simulink model "controller"  (R2024b)
settings: Solver=FixedStepAuto  StartTime=0.0  StopTime=8  FixedStep=0.025  RelTol=1e-3
values from neighbouring files (symbols this model uses):
  DryMass = 3    [FlightPathGeneration.m]
  LaunchSitePressure = PlanMeta(7)    [FlightAnalysis.m]    (also in FlightPathGeneration.m = 101325; TargetApogeeSelection.m = 101325)
  LaunchSiteTemperature = PlanMeta(6)    [FlightAnalysis.m]    (also in FlightPathGeneration.m = 288.15; TargetApogeeSelection.m = 288.15)
  MaximumDragArea = 0.01    [FlightPathGeneration.m]    (also in TargetApogeeSelection.m)
  MinimumDragArea = 0.0025    [FlightPathGeneration.m]    (also in TargetApogeeSelection.m)
undefined symbols (not defined in the file or in its folder): SimAngleSamples, SimMesh, SimVelocitySamples
settings Model: Creator=natha  LastModifiedBy=natha

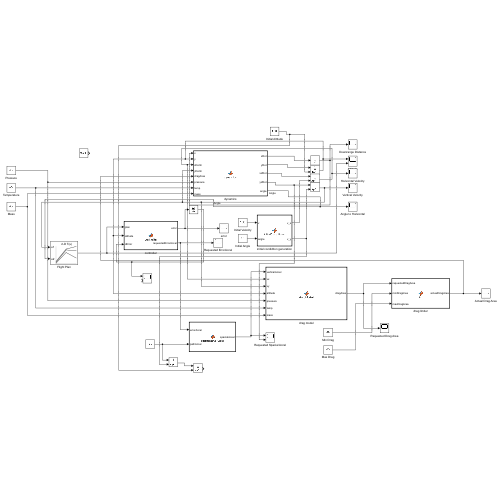
[thumbnail: Simulink's stored preview of the top-level diagram]
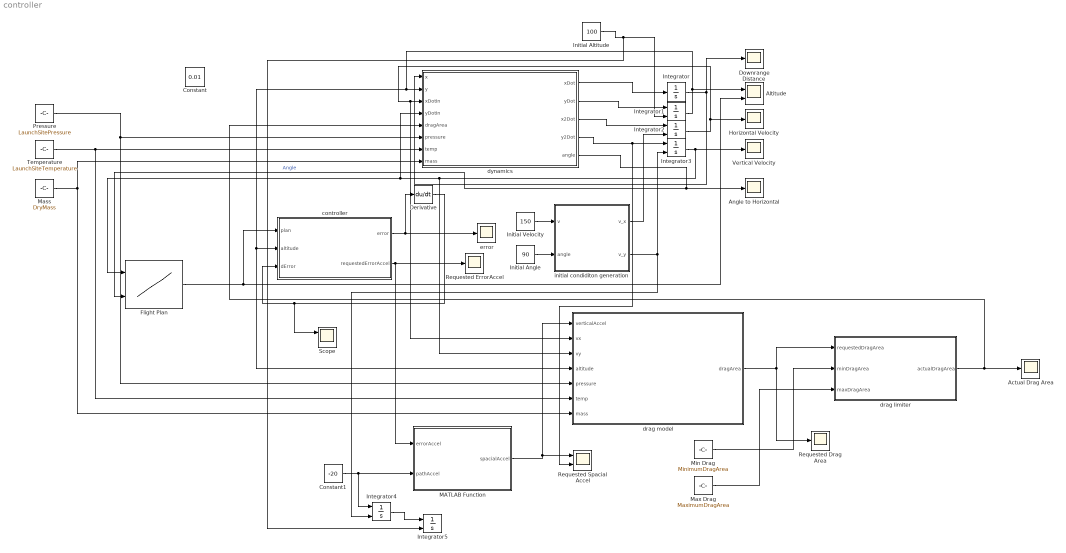
== system controller ==
  Actual Drag Area : Scope
  Altitude : Scope  NumInputPorts=2
  Angle to Horizontal : Scope
  Constant : Constant  Value=0.01
  Constant1 : Constant  Value=-20
  Derivative : Derivative
  Downrange Distance : Scope
  Flight Plan : Lookup_n-D  BreakpointsForDimension1=SimVelocitySamples  BreakpointsForDimension2=SimAngleSamples  Table=SimMesh  InternalRulePriority=Speed  RndMeth=Simplest
      settings: InputPortMap=u0,u1
  Horizontal Velocity : Scope
  Initial Altitude : Constant  Value=100
  Initial Angle : Constant  Value=90
  Initial Velocity : Constant  Value=150
  Integrator : Integrator
  Integrator{1..5} (5 alike) : Integrator  InitialConditionSource=external
  MATLAB Function : MATLAB Function  TreatAsAtomicUnit=on
  Mass : Constant  Value=DryMass
  Max Drag : Constant  Value=MaximumDragArea
  Min Drag : Constant  Value=MinimumDragArea
  Pressure : Constant  Value=LaunchSitePressure
  Requested Drag Area : Scope
  Requested ErrorAccel : Scope
  Requested Spacial Accel : Scope  NumInputPorts=2
  Scope : Scope  NumInputPorts=2
  Temperature : Constant  Value=LaunchSiteTemperature
  Vertical Velocity : Scope
  controller : MATLAB Function  TreatAsAtomicUnit=on
  drag limiter : MATLAB Function  TreatAsAtomicUnit=on
  drag model : MATLAB Function  TreatAsAtomicUnit=on
  dynamics : MATLAB Function  TreatAsAtomicUnit=on
  error : Scope
  initial condiditon generation : MATLAB Function  TreatAsAtomicUnit=on
  wires:
  dynamics/1(xDot) -> Integrator/1
  dynamics/2(yDot) -> Integrator1/1
  dynamics/3(x2Dot) -> Integrator2/1
  dynamics/4(y2Dot) -> Requested Spacial Accel/2, Integrator3/1
  Integrator/1 -> Downrange Distance/1, dynamics/1(x)
  Integrator1/1 -> drag model/4(altitude), controller/2(altitude), dynamics/2(y), Altitude/1
  Integrator2/1 -> drag model/2(vx), dynamics/3(xDotIn), Horizontal Velocity/1
  Integrator3/1 -> Flight Plan/1, dynamics/4(yDotIn), drag model/3(vy), Vertical Velocity/1
  Initial Velocity/1 -> initial condiditon generation/1(v)
  Initial Angle/1 -> initial condiditon generation/2(angle)
  initial condiditon generation/1(v_x) -> Integrator2/2
  initial condiditon generation/2(v_y) -> Integrator3/2, Integrator4/2
  Initial Altitude/1 -> Integrator5/2, Integrator1/2
  dynamics/5(angle) -> Flight Plan/2, Angle to Horizontal/1  "Angle"
  controller/1(error) -> error/1, Derivative/1
  drag model/1(dragArea) -> Requested Drag Area/1, drag limiter/1(requestedDragArea)
  Pressure/1 -> drag model/5(pressure), dynamics/6(pressure)
  Temperature/1 -> drag model/6(temp), dynamics/7(temp)
  drag limiter/1(actualDragArea) -> dynamics/5(dragArea), Actual Drag Area/1
  Mass/1 -> drag model/7(mass), dynamics/8(mass)
  MATLAB Function/1(spacialAccel) -> drag model/1(verticalAccel), Requested Spacial Accel/1
  controller/2(requestedErrorAccel) -> MATLAB Function/1(errorAccel), Requested ErrorAccel/1
  Min Drag/1 -> drag limiter/2(minDragArea)
  Max Drag/1 -> drag limiter/3(maxDragArea)
  Constant1/1 -> Integrator4/1, MATLAB Function/2(pathAccel)
  Integrator4/1 -> Integrator5/1
  Derivative/1 -> Scope/1, controller/3(dError)
  Flight Plan/1 -> Altitude/2, controller/1(plan)

== matlab function controller/initial condiditon generation ==
  data: v input; v_x output; angle input; v_y output
function [v_x, v_y] = initialConditions(v, angle)
v_x = v * cos(angle * pi / 180);
v_y = v * sin(angle * pi / 180);
end

== matlab function controller/dynamics ==
  data: xDot output; yDot output; x2Dot output; y2Dot output; x input; y input; xDotIn input; yDotIn input; dragArea input; angle output; pressure input; temp input; mass input
function [xDot,yDot, x2Dot, y2Dot, angle] = dynamics(x, y, xDotIn, yDotIn, dragArea, pressure, temp, mass)
%constants---
g = 9.8;
%------------
x;
xDot = xDotIn;
yDot = yDotIn;
x2Dot = -1/2/mass * densityFromAltitude(y, pressure, temp) * dragArea * sqrt(xDot * xDot + yDot * yDot) * xDot;
y2Dot = -1/2/mass * densityFromAltitude(y, pressure, temp) * dragArea * sqrt(xDot * xDot + yDot * yDot) * yDot - g;
angle = atan(yDot/xDot);
end


function density = densityFromAltitude(altitude, p0, T0)
    % Constants
    L = 0.0065;      % K/m temperature lapse rate
    g = 9.80665;     % m/s^2 gravitational constant
    R = 8.31446;     % J/(mol*K) Ideal gas constant
    M = 0.0289652;   % kg/mol Molar mass of air
    density = p0*M/(R*T0)*(1-L*altitude/T0).^(g*M/(R*L)-1);
end

== matlab function controller/controller ==
  data: plan input; error output; altitude input; requestedErrorAccel output; dError input
function [error, requestedErrorAccel] = controller(plan, altitude, dError)
%gains
P = -2;
D = -1;
%
error = altitude - plan;
requestedErrorAccel = P*error + D*dError;
end

== matlab function controller/drag model ==
  data: verticalAccel input; dragArea output; vx input; vy input; altitude input; pressure input; temp input; mass input
function dragArea = dragModel(verticalAccel, vx, vy, altitude, pressure, temp, mass)

dragArea = -2 * mass * (verticalAccel) / (densityFromAltitude(altitude,pressure,temp) * sqrt(vx * vx + vy * vy) * vy);
end

function density = densityFromAltitude(altitude, p0, T0)
    % Constants
    L = 0.0065;      % K/m temperature lapse rate
    g = 9.80665;     % m/s^2 gravitational constant
    R = 8.31446;     % J/(mol*K) Ideal gas constant
    M = 0.0289652;   % kg/mol Molar mass of air
    density = p0*M/(R*T0)*(1-L*altitude/T0).^(g*M/(R*L)-1);
end

== matlab function controller/drag limiter ==
  data: requestedDragArea input; actualDragArea output; minDragArea input; maxDragArea input
function actualDragArea = fcn(requestedDragArea, minDragArea, maxDragArea)
if(requestedDragArea > maxDragArea)
    actualDragArea = maxDragArea;
elseif(requestedDragArea< minDragArea)
       actualDragArea = minDragArea;
else
    actualDragArea = requestedDragArea;
end
end

== matlab function controller/MATLAB Function ==
  data: errorAccel input; spacialAccel output; pathAccel input
function spacialAccel = addRelativeAccel(errorAccel, pathAccel)
g = 9.8;
spacialAccel = pathAccel + g + errorAccel;
